simulink model "MRAC_proyecto"  (R2024b)
settings: Solver=ode15s  StartTime=0.0  StopTime=100  RelTol=1e-6
undefined symbols (not defined in the file or in its folder): A_MRAC, Am_MRAC, B_MRAC, Bm_MRAC, C_MRAC, D_MRAC, Gamma_r_MRAC, Gamma_x_MRAC, PB_MRAC, x0_MRAC, xm0_MRAC
settings Model: Creator=juanm  LastModifiedBy=juanm

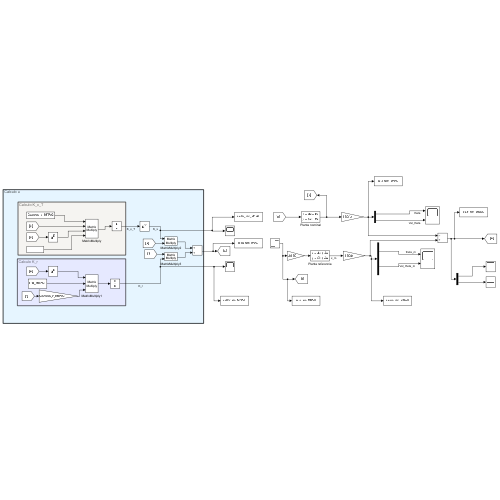
[thumbnail: Simulink's stored preview of the top-level diagram]
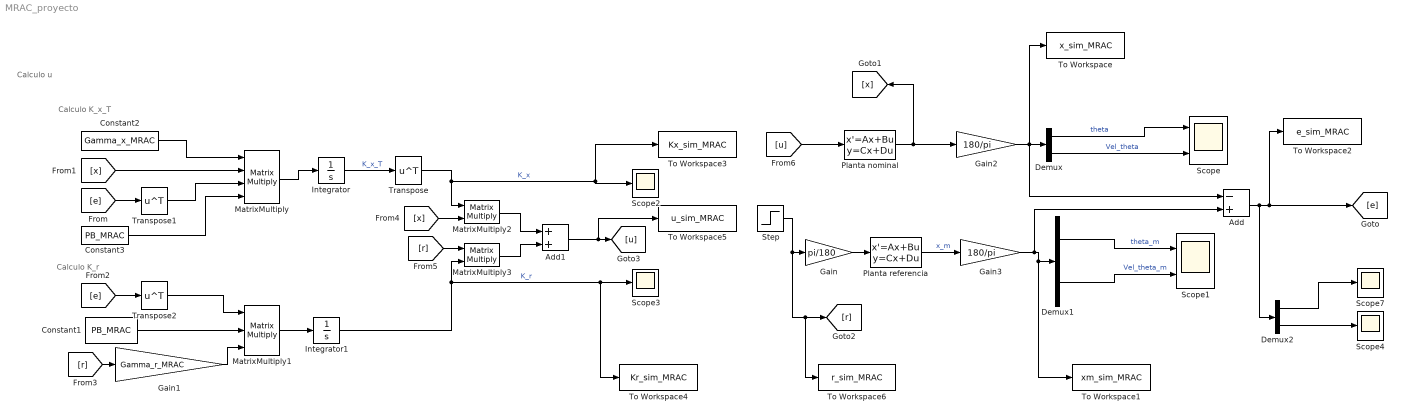
== system MRAC_proyecto ==
  note: Calculo u
  note: Calculo K_r
  note: Calculo K_x_T
  Add : Sum  Inputs=-+
  Add1 : Sum
  Constant1 : Constant  Value=PB_MRAC
  Constant2 : Constant  Value=Gamma_x_MRAC
  Constant3 : Constant  Value=PB_MRAC
  Demux : Demux  Outputs=2
  Demux1 : Demux  Outputs=2
  Demux2 : Demux  Outputs=2
  Gain : Gain  Gain=pi/180
  Gain1 : Gain  Gain=Gamma_r_MRAC
  Gain2 : Gain  Gain=180/pi
  Gain3 : Gain  Gain=180/pi
  Integrator : Integrator  ZeroCross=off
  Integrator1 : Integrator  ZeroCross=off
  MatrixMultiply : Product  Inputs=4  Multiplication=Matrix(*)
  MatrixMultiply1 : Product  Inputs=3  Multiplication=Matrix(*)
  MatrixMultiply2 : Product  Multiplication=Matrix(*)
  MatrixMultiply3 : Product  Multiplication=Matrix(*)
  Planta nominal : StateSpace  A=A_MRAC  B=B_MRAC  C=C_MRAC  D=D_MRAC  InitialCondition=x0_MRAC  ParameterTunability=Unconstrained
  Planta referencia : StateSpace  A=Am_MRAC  B=Bm_MRAC  C=C_MRAC  D=D_MRAC  InitialCondition=xm0_MRAC  ParameterTunability=Unconstrained
  Scope : Scope  NumInputPorts=2
  Scope1 : Scope  NumInputPorts=2
  Scope{2..4,7} (4 alike) : Scope
  Step : Step  After=10  SampleTime=0
  To Workspace : ToWorkspace  VariableName=x_sim_MRAC  SaveFormat=Timeseries  SampleTime=-1
  To Workspace1 : ToWorkspace  VariableName=xm_sim_MRAC  SaveFormat=Timeseries  SampleTime=-1
  To Workspace2 : ToWorkspace  VariableName=e_sim_MRAC  SaveFormat=Timeseries  SampleTime=-1
  To Workspace3 : ToWorkspace  VariableName=Kx_sim_MRAC  SaveFormat=Timeseries  SampleTime=-1
  To Workspace4 : ToWorkspace  VariableName=Kr_sim_MRAC  SaveFormat=Timeseries  SampleTime=-1
  To Workspace5 : ToWorkspace  VariableName=u_sim_MRAC  SaveFormat=Timeseries  SampleTime=-1
  To Workspace6 : ToWorkspace  VariableName=r_sim_MRAC  SaveFormat=Timeseries  SampleTime=-1
  Transpose : Math  Operator=transpose
  Transpose1 : Math  Operator=transpose
  Transpose2 : Math  Operator=transpose
  wires:
  Constant2/1 -> MatrixMultiply/1
  Integrator1/1 -> MatrixMultiply3/2, To Workspace4/1, Scope3/1  "K_r"
  [r] -> Gain1/1
  Constant3/1 -> MatrixMultiply/4
  [u] -> Planta nominal/1
  MatrixMultiply1/1 -> Integrator1/1
  Transpose2/1 -> MatrixMultiply1/1
  [x] -> MatrixMultiply/2
  [x] -> MatrixMultiply2/2
  Planta nominal/1 -> [x], Gain2/1
  Gain1/1 -> MatrixMultiply1/3
  [r] -> MatrixMultiply3/1
  Demux/1 -> Scope/1  "theta"
  Demux1/2 -> Scope1/2  "Vel_theta_m"
  [e] -> Transpose1/1
  Demux/2 -> Scope/2  "Vel_theta"
  Constant1/1 -> MatrixMultiply1/2
  Add/1 -> Demux2/1, To Workspace2/1, [e]
  [e] -> Transpose2/1
  MatrixMultiply/1 -> Integrator/1
  Step/1 -> Gain/1, To Workspace6/1, [r]
  MatrixMultiply3/1 -> Add1/2
  Integrator/1 -> Transpose/1  "K_x_T"
  Transpose/1 -> MatrixMultiply2/1, Scope2/1, To Workspace3/1  "K_x"
  Planta referencia/1 -> Gain3/1  "x_m"
  Demux1/1 -> Scope1/1  "theta_m"
  Transpose1/1 -> MatrixMultiply/3
  Add1/1 -> To Workspace5/1, [u]
  MatrixMultiply2/1 -> Add1/1
  Demux2/1 -> Scope7/1
  Demux2/2 -> Scope4/1
  Gain/1 -> Planta referencia/1
  Gain2/1 -> Add/1, To Workspace/1, Demux/1
  Gain3/1 -> Add/2, To Workspace1/1, Demux1/1
